simulink model "xplane_interface"  (Simulink 7.6)
settings: Solver=FixedStepDiscrete  StartTime=0.0  StopTime=Tfin  FixedStep=Ts  RelTol=1e-3
settings Model: Creator=Borja  LastModifiedBy=frafonal
settings OptimizationCC: InlineParams=on  OptimizeModelRefInitCode=on  LifeSpan=1
settings DebuggingCC: FcnCallInpInsideContextMsg=Enable All
settings RTWCC: SystemTargetFile=ert.tlc  TemplateMakefile=ert_default_tmf  Description=Embedded Coder  ProcessScript=ert_make_rtw_hook
settings CodeAppCC: IgnoreCustomStorageClasses=off
settings ERTTargetCC: MultiwordLength=2048  GenerateSampleERTMain=on  SupportNonFinite=off  InlinedParameterPlacement=NonHierarchical  ERTCustomFileTemplate=example_file_process.tlc  ConvertIfToSwitch=off

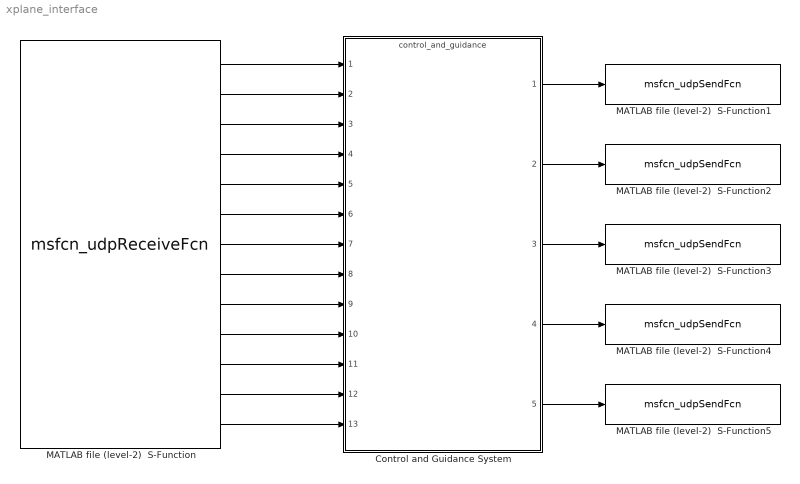
== system xplane_interface ==
  Control and Guidance System : ModelReference  ModelNameDialog=control_and_guidance  SimulationMode=Normal  ModelReferenceVersion=1.458  CopyOfModelName=control_and_guidance  DefaultDataLogging=on
  MATLAB file (level-2)  S-Function : M-S-Function  FunctionName=msfcn_udpReceiveFcn  Parameters=XPLANE_PORT_OUT
      mask Display:
      | port_label('output', 1, 'airspeed')
      | port_label('output', 2, 'pitchRate')
      | port_label('output', 3, 'rollRate')
      | port_label('output', 4, 'yawRate')
      | port_label('output', 5, 'pitch')
      | port_label('output', 6, 'roll')
      | port_label('output', 7, 'heading')
      | port_label('output', 8, 'alpha')
      | port_label('output', 9, 'beta')
      | port_label('output', 10, 'vpath')
      | port_label('output', 11, 'lat')
      | port_label('output', 12, 'lon')
      | port_label('output', 13, 'alt')
      | disp('UDP Receive\n(Java version)')
  MATLAB file (level-2)  S-Function1 : M-S-Function  FunctionName=msfcn_udpSendFcn  Parameters=XPLANE_PORT_IN, XPLANE_IP, dref_elev
      mask Display:
      | port_label('input', 1, 'value')
      | 
      | disp('UDP Send\n(Java version)')
  MATLAB file (level-2)  S-Function2 : M-S-Function  FunctionName=msfcn_udpSendFcn  Parameters=XPLANE_PORT_IN, XPLANE_IP, dref_ailerons
      mask Display:
      | port_label('input', 1, 'value')
      | 
      | disp('UDP Send\n(Java version)')
  MATLAB file (level-2)  S-Function3 : M-S-Function  FunctionName=msfcn_udpSendFcn  Parameters=XPLANE_PORT_IN, XPLANE_IP, dref_rudder
      mask Display:
      | port_label('input', 1, 'value')
      | 
      | disp('UDP Send\n(Java version)')
  MATLAB file (level-2)  S-Function4 : M-S-Function  FunctionName=msfcn_udpSendFcn  Parameters=XPLANE_PORT_IN, XPLANE_IP, dref_engn
      mask Display:
      | port_label('input', 1, 'value')
      | 
      | disp('UDP Send\n(Java version)')
  MATLAB file (level-2)  S-Function5 : M-S-Function  FunctionName=msfcn_udpSendFcn  Parameters=XPLANE_PORT_IN, XPLANE_IP, dref_flaps
      mask Display:
      | port_label('input', 1, 'value')
      | 
      | disp('UDP Send\n(Java version)')
  wires:
  Control and Guidance System/1 -> MATLAB file (level-2)  S-Function1/1
  Control and Guidance System/2 -> MATLAB file (level-2)  S-Function2/1
  Control and Guidance System/3 -> MATLAB file (level-2)  S-Function3/1
  Control and Guidance System/4 -> MATLAB file (level-2)  S-Function4/1
  Control and Guidance System/5 -> MATLAB file (level-2)  S-Function5/1
  MATLAB file (level-2)  S-Function/1 -> Control and Guidance System/1
  MATLAB file (level-2)  S-Function/2 -> Control and Guidance System/2
  MATLAB file (level-2)  S-Function/3 -> Control and Guidance System/3
  MATLAB file (level-2)  S-Function/4 -> Control and Guidance System/4
  MATLAB file (level-2)  S-Function/5 -> Control and Guidance System/5
  MATLAB file (level-2)  S-Function/6 -> Control and Guidance System/6
  MATLAB file (level-2)  S-Function/7 -> Control and Guidance System/7
  MATLAB file (level-2)  S-Function/8 -> Control and Guidance System/8
  MATLAB file (level-2)  S-Function/9 -> Control and Guidance System/9
  MATLAB file (level-2)  S-Function/10 -> Control and Guidance System/10
  MATLAB file (level-2)  S-Function/11 -> Control and Guidance System/11
  MATLAB file (level-2)  S-Function/12 -> Control and Guidance System/12
  MATLAB file (level-2)  S-Function/13 -> Control and Guidance System/13
